simulink subsystem "inverter_switching_variant_closed_loop"  (R2023b)
settings: Solver=VariableStepAuto  StartTime=0.0  StopTime=10.0  RelTol=1e-3
libraries: spsCurrentMeasurementLib x3, spsSeriesRLCBranchLib x2, spsVoltageMeasurementLib x2, spsDCVoltageSourceLib x1, spsGroundLib x1, spsUniversalBridgeLib x1
settings Model: Creator=hwma  LastModifiedBy=hwma

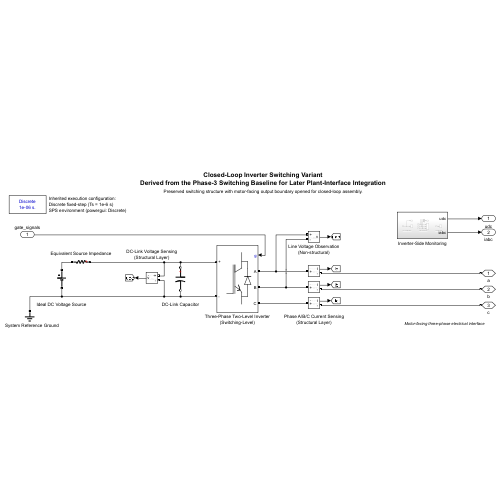
[thumbnail: Simulink's stored preview of the top-level diagram]
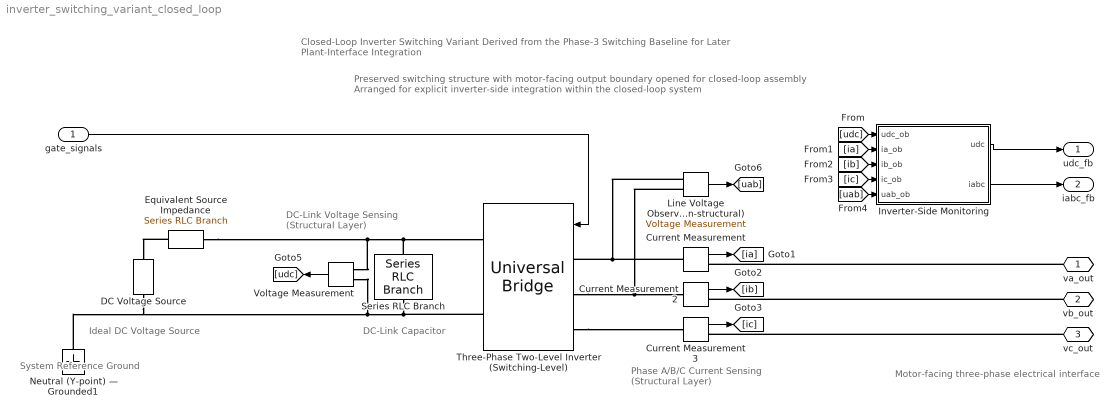
== system inverter_switching_variant_closed_loop ==
  note: Motor-facing three-phase electrical interface
  note: Phase A/B/C Current Sensing
      | (Structural Layer)
  note: DC-Link Capacitor
  note: Ideal DC Voltage Source
  note: Closed-Loop Inverter Switching Variant
      | Derived from the Phase-3 Switching Baseline for Later Plant-Interface Integration
  note: System Reference Ground
  note: DC-Link Voltage Sensing
      | (Structural Layer)
  note: Preserved switching structure with motor-facing output boundary opened for closed-loop assembly
      | Arranged for explicit inverter-side integration within the closed-loop system
  gate_signals : Inport
  Current Measurement : spsCurrentMeasurementLib/Current Measurement  PhasorSimulation=off  OutputType=Complex  PSBequivalent=0
  Current Measurement2 : spsCurrentMeasurementLib/Current Measurement  PhasorSimulation=off  OutputType=Complex  PSBequivalent=0
  Current Measurement3 : spsCurrentMeasurementLib/Current Measurement  PhasorSimulation=off  OutputType=Complex  PSBequivalent=0
  DC Voltage Source : spsDCVoltageSourceLib/DC Voltage Source  Amplitude=800  Measurements=None
  Equivalent Source Impedance : spsSeriesRLCBranchLib/Series RLC Branch  LConnTagsString=__new0  RConnTagsString=__new0  BranchType=R  Resistance=0.01  Inductance=1e-3  SetiL0=off  InitialCurrent=0  Capacitance=1e-6  Setx0=off  InitialVoltage=0  Measurements=None
  Inverter-Side Monitoring : Subsystem
  Line Voltage Observation (Non-structural) : spsVoltageMeasurementLib/Voltage Measurement  PhasorSimulation=off  OutputType=Complex  PSBequivalent=0
  Neutral (Y-point) — Grounded1 : spsGroundLib/Ground  LConnTagsString=a
  Series RLC Branch : spsSeriesRLCBranchLib/Series RLC Branch  LConnTagsString=__new0  RConnTagsString=__new0  BranchType=C  Resistance=1  Inductance=1e-3  SetiL0=off  InitialCurrent=0  Capacitance=1e-3  Setx0=on  InitialVoltage=800  Measurements=None
  Three-Phase Two-Level Inverter (Switching-Level) : spsUniversalBridgeLib/Universal Bridge  Arms=3  SnubberResistance=1e6  SnubberCapacitance=1e-11  Device=IGBT / Diodes  Ron=1e-3  Lon=0  ForwardVoltages="[  0  0  ]"  ForwardVoltage=0  GTOparameters=[ 10e-6 , 20e-6 ]  IGBTparameters=[ 1e-6 , 2e-6 ]  Measurements=None  Measurements_2=None  converterType=Rectifier
  Voltage Measurement : spsVoltageMeasurementLib/Voltage Measurement  PhasorSimulation=off  OutputType=Complex  PSBequivalent=0
  va_out : PMIOPort  Side=Right
  vb_out : PMIOPort  Port=2  Side=Right
  vc_out : PMIOPort  Port=3  Side=Right
  udc_fb : Outport
  iabc_fb : Outport  Port=2
  wires:
  Current Measurement/1 -> [ia]
  Current Measurement2/1 -> [ib]
  gate_signals/1 -> Three-Phase Two-Level Inverter (Switching-Level)/1
  Current Measurement3/1 -> [ic]
  Voltage Measurement/1 -> [udc]
  Line Voltage Observation (Non-structural)/1 -> [uab]
  Inverter-Side Monitoring/2(iabc) -> iabc_fb/1
  Inverter-Side Monitoring/1(udc) -> udc_fb/1
  [udc] -> Inverter-Side Monitoring/1(udc_ob)
  [ia] -> Inverter-Side Monitoring/2(ia_ob)
  [ib] -> Inverter-Side Monitoring/3(ib_ob)
  [ic] -> Inverter-Side Monitoring/4(ic_ob)
  [uab] -> Inverter-Side Monitoring/5(uab_ob)
  connections:
  Line Voltage Observation (Non-structural)/LConn1 -- Current Measurement/LConn1 -- Three-Phase Two-Level Inverter (Switching-Level)/LConn1
  Series RLC Branch/RConn1 -- DC Voltage Source/LConn1 -- Neutral (Y-point) — Grounded1/LConn1 -- Voltage Measurement/LConn2 -- Three-Phase Two-Level Inverter (Switching-Level)/RConn2
  Equivalent Source Impedance/LConn1 -- Three-Phase Two-Level Inverter (Switching-Level)/RConn1 -- Series RLC Branch/LConn1 -- Voltage Measurement/LConn1
  Line Voltage Observation (Non-structural)/LConn2 -- Three-Phase Two-Level Inverter (Switching-Level)/LConn2 -- Current Measurement2/LConn1
  Equivalent Source Impedance/RConn1 -- DC Voltage Source/RConn1
  va_out/RConn1 -- Current Measurement/RConn1
  Three-Phase Two-Level Inverter (Switching-Level)/LConn3 -- Current Measurement3/LConn1
  vb_out/RConn1 -- Current Measurement2/RConn1
  vc_out/RConn1 -- Current Measurement3/RConn1

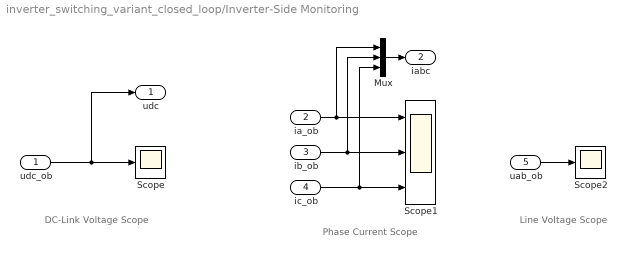
== system inverter_switching_variant_closed_loop/Inverter-Side Monitoring ==
  note: Line Voltage Scope
  note: Phase Current Scope
  note: DC-Link Voltage Scope
  udc_ob : Inport
  ia_ob : Inport  Port=2
  ib_ob : Inport  Port=3
  ic_ob : Inport  Port=4
  uab_ob : Inport  Port=5
  Mux : Mux  Inputs=3
  Scope : Scope
  Scope1 : Scope  NumInputPorts=3
  Scope2 : Scope
  udc : Outport
  iabc : Outport  Port=2
  wires:
  Mux/1 -> iabc/1
  uab_ob/1 -> Scope2/1
  ic_ob/1 -> Scope1/3, Mux/3
  ib_ob/1 -> Scope1/2, Mux/2
  ia_ob/1 -> Scope1/1, Mux/1
  udc_ob/1 -> Scope/1, udc/1
